simulink model "RobotModel"  (R2019a)
settings: Solver=VariableStepAuto  StartTime=0.0  StopTime=100  RelTol=1e-3
InitFcn:
  | robotInit
StopFcn:
  | SLAMmap
model workspace (MAT data in the model file):
  MCOS : class17 (value not decoded)
  MCOS : class17 (value not decoded)
values from neighbouring files (symbols this model uses):
  b = 0.5    [neuraldata.mat]    (also in robotInit.m)
  behavior = 0    [neuraldata.mat]    (also in robotInit.m)
  goal_pos = [15 10]    [neuraldata.mat]    (also in robotInit.m = [20;30])
  min_obs_dist = 0.5    [neuraldata.mat]    (also in robotInit.m)
  P = (eye(size(K,1))-K*H)*P    [extKalmanFilter.m]    (also in neuraldata.mat = [0 0 0 0 0 0 0 0 0 0 0 0 ... (25 elements, 5x5)]; robotInit.m = zeros(5,5))
  Q = diag([0 0 0 0 0])    [extKalmanFilter.m]    (also in neuraldata.mat = [0 0 0 0 0 0 0 0 0 0 0 0 ... (25 elements, 5x5)]; robotInit.m = diag([0 0 0 0.5 0.5]))
  R = 0.005/Ts    (= 0.1)    [extKalmanFilter.m]    (also in neuraldata.mat = [0.1 0 0 0 0 0.1 0 0 0 0 0.5 0 ... (16 elements, 4x4)]; robotInit.m = diag([0.1 0.1 0.5 0.5]))
  r = 0.1    [neuraldata.mat]    (also in robotInit.m)
  sense_angles = 0:(pi/20):2*pi    [SLAMmap.m]    (also in neuraldata.mat = [0 0.157079632679 0.314159265359 0.471238898038 0.6283185307; robotInit.m = 0:(pi/20):(2*pi))
  start_pos = [20 30 0]    [neuraldata.mat]    (also in robotInit.m = [5;5;0])
  Ts = 0.05    [extKalmanFilter.m]    (also in gpsMeasurementFcn.m; neuraldata.mat; robotInit.m)
  xhat = xhat + K*resid    [extKalmanFilter.m]    (also in neuraldata.mat = [20 30 0 0 0]; robotInit.m = [start_pos;0;0])
undefined symbols (not defined in the file or in its folder): robot_pose
libraries: neural x60, mobileRoboticsLib x7
(part 3 of 3)

== matlab function RobotModel/Subsystem/MATLAB Function4 ==
  data: P input; r output; Q input; sigp input; sigt input; robot_pos input; a output; covM output; x_line output; y_line output
function [r,a,covM,x_line,y_line]=inc_line_extract(P, Q,sigp,sigt,robot_pos)

n = length(P);
x_line=[];
y_line=[];

x=robot_pos(1);
y=robot_pos(2);
th=robot_pos(3);
R=[cos(th) -sin(th); sin(th) cos(th)];

%thresholds for classifying lines as the same
r_thresh=.25;
a_thresh=.01;

%Extract First Line
[r_temp,a_temp,covM_temp]=compute_line_params(P(1:2),Q(1:2),sigp,sigt);
i_start=1;
line_count=0;
i=3;

if n<3
    r=r_temp;
    a=a_temp;
    covM=covM_temp;
    [xline_temp,yline_temp]=compute_ra_line(r,a,P(1),Q(1),P(2),Q(2));
    xy_temp=[x x;y y]+R*[xline_temp;yline_temp];
    
    x_line=[x_line,xy_temp(1,:)];
    y_line=[y_line,xy_temp(2,:)];
end

while i <= n
    
    [r_temp2,a_temp2,covM_temp2]=compute_line_params(P(i_start:i),Q(i_start:i),sigp,sigt);
    
    %time to split, point i didn't work
    if abs(1-r_temp2/r_temp)>r_thresh || abs(a_temp-a_temp2)>a_thresh
        line_count=line_count+1;
        r(line_count)=r_temp;
        a(line_count)=a_temp;
        covM{line_count}=covM_temp;
        %%%%%%%%%%%%%%%%%%%%%%%%%%%%%%%%%%%%%%%%%%%%%%%%%%%%%%%%%%%%%%%
        %Plotting Purposes Only
        %%%%%%%%%%%%%%%%%%%%%%%%%%%%%%%%%%%%%%%%%%%%%%%%%%%%%%%%%%%%%%%
        [xline_temp,yline_temp]=compute_ra_line(r(line_count),a(line_count),P(i_start),Q(i_start),P(i-1),Q(i-1));

        xy_temp=[x x;y y]+R*[xline_temp;yline_temp];
        
        x_line=[x_line,xy_temp(1,:)];
        y_line=[y_line,xy_temp(2,:)];
        %%%%%%%%%%%%%%%%%%%%%%%%%%%%%%%%%%%%%%%%%%%%%%%%%%%%%%%%%%%%%%%
        i_start=i-1;
        
        [r_temp,a_temp,covM_temp]=compute_line_params(P(i_start:i),Q(i_start:i),sigp,sigt);
        
    else  %lines are the same, goto next point
        r_temp=r_temp2;
        a_temp=a_temp2;
        covM_temp=covM_temp2;
        
        %last point in scan, save line
        if i==n
            line_count=line_count+1;
            r(line_count)=r_temp;
            a(line_count)=a_temp;
            covM{line_count}=covM_temp;
            %%%%%%%%%%%%%%%%%%%%%%%%%%%%%%%%%%%%%%%%%%%%%%%%%%%%%%%%%%%%%%%
            %Plotting Purposes Only
            %%%%%%%%%%%%%%%%%%%%%%%%%%%%%%%%%%%%%%%%%%%%%%%%%%%%%%%%%%%%%%%
            [xline_temp,yline_temp]=compute_ra_line(r(line_count),a(line_count),P(i_start),Q(i_start),P(end),Q(end));

            xy_temp=[x x;y y]+R*[xline_temp;yline_temp];
            
            x_line=[x_line,xy_temp(1,:)];
            y_line=[y_line,xy_temp(2,:)];
            %%%%%%%%%%%%%%%%%%%%%%%%%%%%%%%%%%%%%%%%%%%%%%%%%%%%%%%%%%%%%%%
        end
    end
    i=i+1;
end

== matlab function RobotModel/Subsystem/MATLAB Function5 ==
  data: pose input; gps_coord output
function gps_coord = gpsGenerate(pose)
sigma = 0.1;
coder.extrinsic('rand')
x = pose(1);
y = pose(2);
xNoise = x + (sqrt(sigma)*randn);
yNoise = y + (sqrt(sigma)*randn);
gps_coord = [xNoise; yNoise];

== matlab function RobotModel/Subsystem/MATLAB Function6 ==
  data: in input; meas input; pose output; vel output; Pin input; Rin input; Qin input; Ts input; xhatin input
function [pose, vel] = extKalmanFilter(in, meas, Pin, Rin, Qin, Ts, xhatin)
persistent P R Q xhat
if isempty(P)
P = Pin; R = Rin; Q = Qin; xhat= xhatin;
end

F = [1 0 0 Ts*cos(xhat(3)+Ts*xhat(5)/2) 0;
     0 1 0 Ts*sin(xhat(3)+Ts*xhat(5)/2) 0;
     0 0 1 0 Ts;
     0 0 0 1 0;
     0 0 0 0 1];
 
H = [1 0 0 0 0; 0 1 0 0 0; 0 0 0 1 0; 0 0 0 0 1];
xhat = [(xhat(1) + xhat(4)*(Ts)*cos(xhat(3)+Ts*xhat(5)/2));
        (xhat(2) + xhat(4)*(Ts)*sin(xhat(3)+Ts*xhat(5)/2));
        (xhat(3) + Ts*xhat(5));
        (sign(xhat(4))*in(1));
        (sign(xhat(5))*in(2))];
P = F*P*F' + Q;
% Calculate the Kalman gain
K = P*H'/(H*P*H' + R);
% Calculate the measurement residual
yhat = [xhat(1);xhat(2);xhat(4);xhat(5)];
resid = meas - yhat;
% Update the state and covariance estimates
xhat = xhat + K*resid;
P = (eye(size(K,1))-K*H)*P;
% Post the results
pose = [xhat(1);xhat(2);xhat(3)];
vel = [xhat(4);xhat(5)];

== matlab function RobotModel/Subsystem/MATLAB Function7 ==
  data: A input; meas output; B input
function meas = fuseSensorInput(A, B)
meas = [B(1);B(2);A(1);A(2)];
end
